simulink model "LQDG_Pitch"  (R2020a)
settings: Solver=ode3  StartTime=0.0  StopTime=inf  FixedStep=0.01  RelTol=1e-3  EnableMultiTasking=on
values from neighbouring files (symbols this model uses):
  LQDG_gain = R1_inv*B'*k1_ans    [untitled2.m]
  weighting_matrix = XOpt    [load_data.m]
undefined symbols (not defined in the file or in its folder): B1, B3, rad, s
libraries: arduinolib x5, aerolibconvert2 x4
settings Model: SILPILModeSetting=veronly  ExtModeTrigDuration=2  Creator=Ali  LastModifiedBy=Ali
settings OptimizationCC: EnhancedBackFolding=on  PassReuseOutputArgsAs=Individual arguments  ZeroExternalMemoryAtStartup=off  ZeroInternalMemoryAtStartup=off  MaxStackSize=64  OptimizeBlockOrder=speed  DifferentSizesBufferReuse=on  OptimizationCustomize=off  EfficientTunableParamExpr=on
settings DebuggingCC: ParameterTunabilityLossMsg=error
settings HardwareCC: ProdBitPerInt=16  ProdBitPerPointer=16  ProdBitPerSizeT=16  ProdBitPerPtrDiffT=16  ProdLargestAtomicFloat=None  ProdWordSize=8  ProdHWDeviceType=Atmel->AVR
settings SFSimCC: MATLABDynamicMemAlloc=off
settings RTWCC: SystemTargetFile=ert.tlc  HardwareBoard=Arduino Mega 2560  TLCOptions=-aInlineSetEventsForThisBaseRateFcn=TLC_FALSE -aSuppressMultiTaskScheduler=TLC_FALSE -aRateBasedStepFcn=1  TemplateMakefile=ert_default_tmf  Toolchain=Arduino AVR  BuildConfiguration=Faster Runs
settings CodeAppCC: ForceParamTrailComments=on  IgnoreCustomStorageClasses=off  OperatorAnnotations=on  SimulinkDataObjDesc=on  SFDataObjDesc=on  InsertBlockDesc=on
settings ERTTargetCC: SupportContinuousTime=on  SupportVariableSizeSignals=on  ExtModeStaticAllocSize=2048

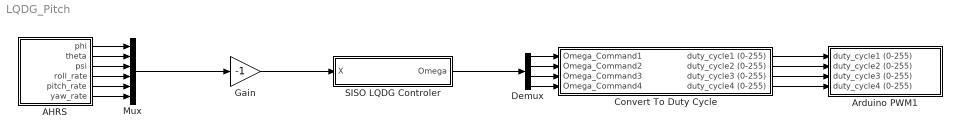
== system LQDG_Pitch ==
  AHRS : Subsystem
  Arduino PWM1 : Subsystem  mask{Motor1=8, Motor2=9, Motor3=10, Motor4=11}
      mask prompts: Motor1 "Motor 1 Pin Number"; Motor2 "Motor 2 Pin Number"; Motor3 "Motor 3 Pin Number"; Motor4 "Motor 4 Pin Number"
  Convert To Duty Cycle : Subsystem
  Demux : Demux
  Gain : Gain  Gain=-1
  Mux : Mux  Inputs=6
  SISO LQDG Controler : Subsystem
  wires:
  Convert To Duty Cycle/3(duty_cycle3 (0-255)) -> Arduino PWM1/3(duty_cycle3 (0-255))
  Convert To Duty Cycle/1(duty_cycle1 (0-255)) -> Arduino PWM1/1(duty_cycle1 (0-255))
  Convert To Duty Cycle/4(duty_cycle4 (0-255)) -> Arduino PWM1/4(duty_cycle4 (0-255))
  Convert To Duty Cycle/2(duty_cycle2 (0-255)) -> Arduino PWM1/2(duty_cycle2 (0-255))
  Demux/1 -> Convert To Duty Cycle/1(Omega_Command1)
  Demux/2 -> Convert To Duty Cycle/2(Omega_Command2)
  Demux/3 -> Convert To Duty Cycle/3(Omega_Command3)
  Demux/4 -> Convert To Duty Cycle/4(Omega_Command4)
  AHRS/1(phi) -> Mux/1
  AHRS/2(theta) -> Mux/2
  AHRS/3(psi) -> Mux/3
  AHRS/4(roll_rate) -> Mux/4
  AHRS/5(pitch_rate) -> Mux/5
  AHRS/6(yaw_rate) -> Mux/6
  Gain/1 -> SISO LQDG Controler/1(X)
  SISO LQDG Controler/1(Omega) -> Demux/1
  Mux/1 -> Gain/1

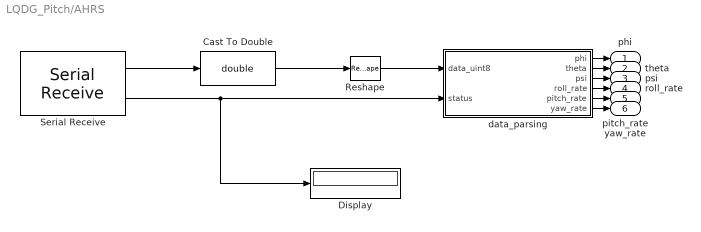
== system LQDG_Pitch/AHRS ==
  Cast To Double : DataTypeConversion  OutDataTypeStr=double
  Display : Display
  Reshape : Reshape
  Serial Receive : arduinolib/Serial Receive  isARMArch=off  portNumber=1  DataType=uint8  Datalength=32  SampleTime=0.01  showOutStatus=on  blockPlatform=arduino
      settings: SourceProductBaseCode=ARDUINO
  data_parsing : MATLAB Function  TreatAsAtomicUnit=on
  phi : Outport
  theta : Outport  Port=2
  psi : Outport  Port=3
  roll_rate : Outport  Port=4
  pitch_rate : Outport  Port=5
  yaw_rate : Outport  Port=6
  wires:
  data_parsing/2(theta) -> theta/1
  data_parsing/3(psi) -> psi/1
  data_parsing/4(roll_rate) -> roll_rate/1
  Reshape/1 -> data_parsing/1(data_uint8)
  data_parsing/1(phi) -> phi/1
  data_parsing/5(pitch_rate) -> pitch_rate/1
  Serial Receive/2 -> Display/1, data_parsing/2(status)
  data_parsing/6(yaw_rate) -> yaw_rate/1
  Cast To Double/1 -> Reshape/1
  Serial Receive/1 -> Cast To Double/1

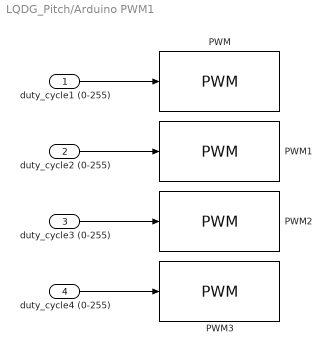
== system LQDG_Pitch/Arduino PWM1 ==
  duty_cycle1 (0-255) : Inport
  duty_cycle2 (0-255) : Inport  Port=2
  duty_cycle3 (0-255) : Inport  Port=3
  duty_cycle4 (0-255) : Inport  Port=4
  PWM : arduinolib/PWM  pinNumber=Motor1  frequencyType=Default  desiredFrequency=490.2  achievableFrequency=490.2
  PWM1 : arduinolib/PWM  pinNumber=Motor2  frequencyType=Default  desiredFrequency=490.2  achievableFrequency=490.2
  PWM2 : arduinolib/PWM  pinNumber=Motor3  frequencyType=Default  desiredFrequency=490.2  achievableFrequency=490.2
  PWM3 : arduinolib/PWM  pinNumber=Motor4  frequencyType=Default  desiredFrequency=490.2  achievableFrequency=490.2
  wires:
  duty_cycle1 (0-255)/1 -> PWM/1
  duty_cycle2 (0-255)/1 -> PWM1/1
  duty_cycle3 (0-255)/1 -> PWM2/1
  duty_cycle4 (0-255)/1 -> PWM3/1

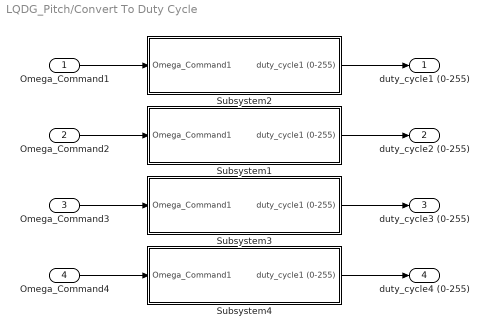
== system LQDG_Pitch/Convert To Duty Cycle ==
  Omega_Command1 : Inport
  Omega_Command2 : Inport  Port=2
  Omega_Command3 : Inport  Port=3
  Omega_Command4 : Inport  Port=4
  Subsystem1 : Subsystem
  Subsystem2 : Subsystem
  Subsystem3 : Subsystem
  Subsystem4 : Subsystem
  duty_cycle1 (0-255) : Outport
  duty_cycle2 (0-255) : Outport  Port=2
  duty_cycle3 (0-255) : Outport  Port=3
  duty_cycle4 (0-255) : Outport  Port=4
  wires:
  Subsystem1/1(duty_cycle1 (0-255)) -> duty_cycle2 (0-255)/1
  Subsystem3/1(duty_cycle1 (0-255)) -> duty_cycle3 (0-255)/1
  Subsystem4/1(duty_cycle1 (0-255)) -> duty_cycle4 (0-255)/1
  Subsystem2/1(duty_cycle1 (0-255)) -> duty_cycle1 (0-255)/1
  Omega_Command1/1 -> Subsystem2/1(Omega_Command1)
  Omega_Command4/1 -> Subsystem4/1(Omega_Command1)
  Omega_Command3/1 -> Subsystem3/1(Omega_Command1)
  Omega_Command2/1 -> Subsystem1/1(Omega_Command1)

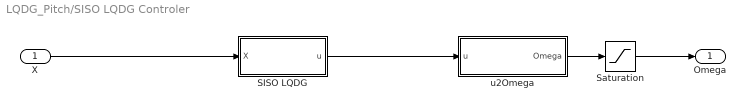
== system LQDG_Pitch/SISO LQDG Controler ==
  X : Inport
  SISO LQDG : Subsystem
  Saturation : Saturate  UpperLimit=6000*2*pi/60  LowerLimit=1500*2*pi/60
  u2Omega : Subsystem
  Omega : Outport
  wires:
  X/1 -> SISO LQDG/1(X)
  SISO LQDG/1(u) -> u2Omega/1(u)
  u2Omega/1(Omega) -> Saturation/1
  Saturation/1 -> Omega/1

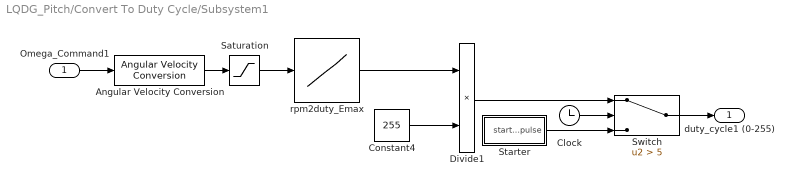
== system LQDG_Pitch/Convert To Duty Cycle/Subsystem1 ==
  Omega_Command1 : Inport
  Angular Velocity Conversion : aerolibconvert2/Angular Velocity Conversion  IU=rad/s  OU=rpm
  Clock : Clock
  Constant4 : Constant  Value=255
  Divide1 : Product  Inputs=**
  Saturation : Saturate  UpperLimit=6000  LowerLimit=1300
  Starter : Subsystem
  Switch : Switch  Criteria=u2 > Threshold  Threshold=5
  rpm2duty_Emax : Lookup_n-D  NumberOfTableDimensions=1  BreakpointsForDimension1=|  Table=|  RndMeth=Simplest  InputSameDT=on
      BreakpointsForDimension1=|
      | [1201
      | 2305
      | 3096
      | 3930
      | 4118
      | 4555
      | 5122
      | 5552
      | 5957
      | 6291
      | 6360]
      Table=|
      | [0.5
      | 0.55
      | 0.6
      | 0.65
      | 0.7
      | 0.75
      | 0.8
      | 0.85
      | 0.9
      | 0.95
      | 1]
  duty_cycle1 (0-255) : Outport
  wires:
  Divide1/1 -> Switch/1
  Switch/1 -> duty_cycle1 (0-255)/1
  Clock/1 -> Switch/2
  Starter/1(start_pulse) -> Switch/3
  Angular Velocity Conversion/1 -> Saturation/1
  Constant4/1 -> Divide1/2
  Omega_Command1/1 -> Angular Velocity Conversion/1
  rpm2duty_Emax/1 -> Divide1/1
  Saturation/1 -> rpm2duty_Emax/1

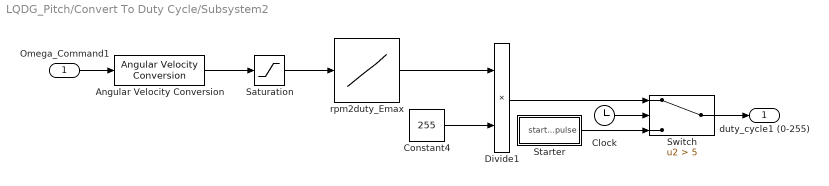
== system LQDG_Pitch/Convert To Duty Cycle/Subsystem2 ==
  Omega_Command1 : Inport
  Angular Velocity Conversion : aerolibconvert2/Angular Velocity Conversion  IU=rad/s  OU=rpm
  Clock : Clock
  Constant4 : Constant  Value=255
  Divide1 : Product  Inputs=**
  Saturation : Saturate  UpperLimit=6000  LowerLimit=1300
  Starter : Subsystem
  Switch : Switch  Criteria=u2 > Threshold  Threshold=5
  rpm2duty_Emax : Lookup_n-D  NumberOfTableDimensions=1  BreakpointsForDimension1=|  Table=|  RndMeth=Simplest  InputSameDT=on
      BreakpointsForDimension1=|
      | [1201
      | 2305
      | 3096
      | 3930
      | 4118
      | 4555
      | 5122
      | 5552
      | 5957
      | 6291
      | 6360]
      Table=|
      | [0.5
      | 0.55
      | 0.6
      | 0.65
      | 0.7
      | 0.75
      | 0.8
      | 0.85
      | 0.9
      | 0.95
      | 1]
  duty_cycle1 (0-255) : Outport
  wires:
  Omega_Command1/1 -> Angular Velocity Conversion/1
  Constant4/1 -> Divide1/2
  Angular Velocity Conversion/1 -> Saturation/1
  Starter/1(start_pulse) -> Switch/3
  Clock/1 -> Switch/2
  Switch/1 -> duty_cycle1 (0-255)/1
  Divide1/1 -> Switch/1
  rpm2duty_Emax/1 -> Divide1/1
  Saturation/1 -> rpm2duty_Emax/1

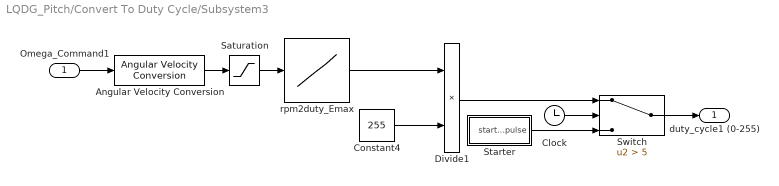
== system LQDG_Pitch/Convert To Duty Cycle/Subsystem3 ==
  Omega_Command1 : Inport
  Angular Velocity Conversion : aerolibconvert2/Angular Velocity Conversion  IU=rad/s  OU=rpm
  Clock : Clock
  Constant4 : Constant  Value=255
  Divide1 : Product  Inputs=**
  Saturation : Saturate  UpperLimit=6000  LowerLimit=1300
  Starter : Subsystem
  Switch : Switch  Criteria=u2 > Threshold  Threshold=5
  rpm2duty_Emax : Lookup_n-D  NumberOfTableDimensions=1  BreakpointsForDimension1=|  Table=|  RndMeth=Simplest  InputSameDT=on
      BreakpointsForDimension1=|
      | [1201
      | 2305
      | 3096
      | 3930
      | 4118
      | 4555
      | 5122
      | 5552
      | 5957
      | 6291
      | 6360]
      Table=|
      | [0.5
      | 0.55
      | 0.6
      | 0.65
      | 0.7
      | 0.75
      | 0.8
      | 0.85
      | 0.9
      | 0.95
      | 1]
  duty_cycle1 (0-255) : Outport
  wires:
  Omega_Command1/1 -> Angular Velocity Conversion/1
  Constant4/1 -> Divide1/2
  Angular Velocity Conversion/1 -> Saturation/1
  Starter/1(start_pulse) -> Switch/3
  Clock/1 -> Switch/2
  Switch/1 -> duty_cycle1 (0-255)/1
  Divide1/1 -> Switch/1
  rpm2duty_Emax/1 -> Divide1/1
  Saturation/1 -> rpm2duty_Emax/1

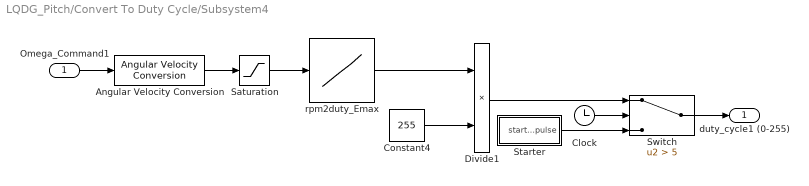
== system LQDG_Pitch/Convert To Duty Cycle/Subsystem4 ==
  Omega_Command1 : Inport
  Angular Velocity Conversion : aerolibconvert2/Angular Velocity Conversion  IU=rad/s  OU=rpm
  Clock : Clock
  Constant4 : Constant  Value=255
  Divide1 : Product  Inputs=**
  Saturation : Saturate  UpperLimit=6000  LowerLimit=1300
  Starter : Subsystem
  Switch : Switch  Criteria=u2 > Threshold  Threshold=5
  rpm2duty_Emax : Lookup_n-D  NumberOfTableDimensions=1  BreakpointsForDimension1=|  Table=|  RndMeth=Simplest  InputSameDT=on
      BreakpointsForDimension1=|
      | [1201
      | 2305
      | 3096
      | 3930
      | 4118
      | 4555
      | 5122
      | 5552
      | 5957
      | 6291
      | 6360]
      Table=|
      | [0.5
      | 0.55
      | 0.6
      | 0.65
      | 0.7
      | 0.75
      | 0.8
      | 0.85
      | 0.9
      | 0.95
      | 1]
  duty_cycle1 (0-255) : Outport
  wires:
  Divide1/1 -> Switch/1
  Switch/1 -> duty_cycle1 (0-255)/1
  Clock/1 -> Switch/2
  Starter/1(start_pulse) -> Switch/3
  Angular Velocity Conversion/1 -> Saturation/1
  Constant4/1 -> Divide1/2
  Omega_Command1/1 -> Angular Velocity Conversion/1
  rpm2duty_Emax/1 -> Divide1/1
  Saturation/1 -> rpm2duty_Emax/1

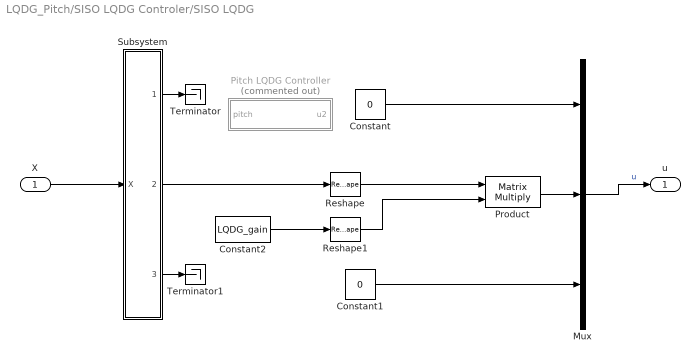
== system LQDG_Pitch/SISO LQDG Controler/SISO LQDG ==
  X : Inport
  Constant : Constant  Value=0
  Constant1 : Constant  Value=0
  Constant2 : Constant  Value=LQDG_gain
  Mux : Mux  Inputs=3
  Pitch LQDG Controller : Subsystem  Commented=on
  Product : Product  Multiplication=Matrix(*)
  Reshape : Reshape  OutputDimensionality=Row vector (2-D)
  Reshape1 : Reshape  OutputDimensionality=Column vector (2-D)
  Subsystem : Subsystem
  Terminator : Terminator
  Terminator1 : Terminator
  u : Outport
  wires:
  Mux/1 -> u/1  "u"
  X/1 -> Subsystem/1(X)
  Subsystem/1(roll) -> Terminator/1
  Constant/1 -> Mux/1
  Subsystem/3(yaw) -> Terminator1/1
  Constant1/1 -> Mux/3
  Subsystem/2(pitch) -> Reshape/1
  Constant2/1 -> Reshape1/1
  Reshape/1 -> Product/1
  Product/1 -> Mux/2
  Reshape1/1 -> Product/2

== system LQDG_Pitch/SISO LQDG Controler/u2Omega ==
  u : Inport
  MATLAB Function1 : MATLAB Function  TreatAsAtomicUnit=on
  Mux1 : Mux
  Omega : Outport
  wires:
  Mux1/1 -> Omega/1
  MATLAB Function1/2(omega_2) -> Mux1/2
  u/1 -> MATLAB Function1/1(u)
  MATLAB Function1/3(omega_3) -> Mux1/3
  MATLAB Function1/1(omega_1) -> Mux1/1
  MATLAB Function1/4(omega_4) -> Mux1/4

== system LQDG_Pitch/Convert To Duty Cycle/Subsystem1/Starter ==
  Add : Sum
  Step : Step  After=140
  Step1 : Step  Time=2  After=-30
  start_pulse : Outport
  wires:
  Add/1 -> start_pulse/1
  Step/1 -> Add/1
  Step1/1 -> Add/2

== system LQDG_Pitch/Convert To Duty Cycle/Subsystem2/Starter ==
  Add : Sum
  Step : Step  After=140
  Step1 : Step  Time=2  After=-30
  start_pulse : Outport
  wires:
  Add/1 -> start_pulse/1
  Step/1 -> Add/1
  Step1/1 -> Add/2

== system LQDG_Pitch/Convert To Duty Cycle/Subsystem3/Starter ==
  Add : Sum
  Step : Step  After=140
  Step1 : Step  Time=2  After=-30
  start_pulse : Outport
  wires:
  Add/1 -> start_pulse/1
  Step/1 -> Add/1
  Step1/1 -> Add/2

== system LQDG_Pitch/Convert To Duty Cycle/Subsystem4/Starter ==
  Add : Sum
  Step : Step  After=140
  Step1 : Step  Time=2  After=-30
  start_pulse : Outport
  wires:
  Add/1 -> start_pulse/1
  Step/1 -> Add/1
  Step1/1 -> Add/2

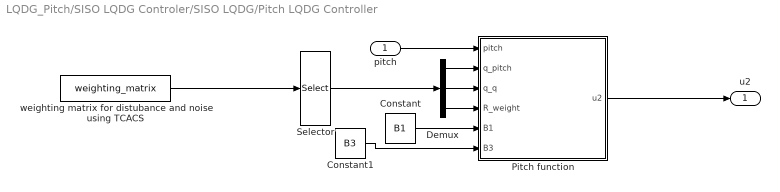
== system LQDG_Pitch/SISO LQDG Controler/SISO LQDG/Pitch LQDG Controller ==
  pitch : Inport
  Constant : Constant  Value=B1
  Constant1 : Constant  Value=B3
  Demux : Demux  Outputs=3
  Pitch function : MATLAB Function  TreatAsAtomicUnit=on
  Selector : Selector  InputPortWidth=5  IndexOptions=Index vector (dialog)  Indices=[1 3 5]  OutputSizes=1
  weighting matrix for distubance and noise using TCACS : Constant  Value=weighting_matrix
  u2 : Outport
  wires:
  Pitch function/1(u2) -> u2/1
  Demux/1 -> Pitch function/2(q_pitch)
  Demux/3 -> Pitch function/4(R_weight)
  Selector/1 -> Demux/1
  Demux/2 -> Pitch function/3(q_q)
  weighting matrix for distubance and noise using TCACS/1 -> Selector/1
  pitch/1 -> Pitch function/1(pitch)
  Constant/1 -> Pitch function/5(B1)
  Constant1/1 -> Pitch function/6(B3)

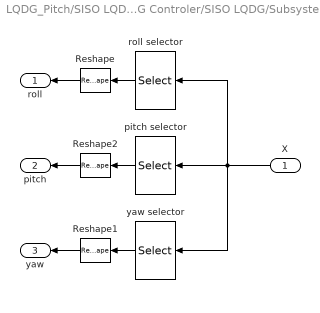
== system LQDG_Pitch/SISO LQDG Controler/SISO LQDG/Subsystem ==
  X : Inport
  Reshape : Reshape  OutputDimensionality=Column vector (2-D)
  Reshape1 : Reshape  OutputDimensionality=Column vector (2-D)
  Reshape2 : Reshape  OutputDimensionality=Column vector (2-D)
  pitch selector : Selector  InputPortWidth=6  IndexOptions=Index vector (dialog)  Indices=[2 5]  OutputSizes=1
  roll selector : Selector  InputPortWidth=6  IndexOptions=Index vector (dialog)  Indices=[1 4]  OutputSizes=1
  yaw selector : Selector  InputPortWidth=6  IndexOptions=Index vector (dialog)  Indices=[3 6]  OutputSizes=1
  roll : Outport
  pitch : Outport  Port=2
  yaw : Outport  Port=3
  wires:
  X/1 -> yaw selector/1, roll selector/1, pitch selector/1
  roll selector/1 -> Reshape/1
  pitch selector/1 -> Reshape2/1
  yaw selector/1 -> Reshape1/1
  Reshape/1 -> roll/1
  Reshape2/1 -> pitch/1
  Reshape1/1 -> yaw/1

== matlab function LQDG_Pitch/SISO LQDG Controler/u2Omega/MATLAB Function1 ==
  data: u input size=3; omega_1 output size=1; omega_2 output size=1; omega_3 output size=1; omega_4 output size=1
function [omega_1, omega_2, omega_3, omega_4] = fcn(u)
u1 = u(1);
u2 = u(2);
u3 = u(3);
% control effort
u4 = ones(1, length(u1)) * 4 * rpm2rad_sec(2000)^2;
% calculate omega
if (u4 + u3 + 2 * u2) / 4 > 0
    omega_1 = sqrt((u4 + u3 + 2 * u2) / 4);
else
    omega_1 = 0;
end
if (u4 + u3 - 2 * u2) / 4 > 0
    omega_3 = sqrt((u4 + u3 - 2 * u2) / 4);
else
    omega_3 = 0;
end
if (u4 - u3 + 2 * u1) / 4 > 0
    omega_2 = sqrt((u4 - u3 + 2 * u1) / 4);
else
    omega_2 = 0;
end
if (u4 - u3 - 2 * u1) / 4 > 0
    omega_4 = sqrt((u4 - u3 - 2 * u1) / 4);
else
    omega_4 = 0;
end
end
%% functions
% rpm to rad/sec
function rad = rpm2rad_sec(rpm)
rad = rpm / 60 * 2 * pi;
end

== matlab function LQDG_Pitch/AHRS/data_parsing ==
  data: phi output size=1; data_uint8 input size=32; theta output size=1; psi output size=1; roll_rate output size=1; pitch_rate output size=1; yaw_rate output size=1; status input
function [phi,theta,psi,roll_rate,pitch_rate,yaw_rate] = fcn(data_uint8, status)
persistent stepp check_sum...
    phi_p theta_p psi_p roll_rate_p pitch_rate_p yaw_rate_p...
    phi_last theta_last psi_last roll_rate_last pitch_rate_last yaw_rate_last;
%% Initialize
if isempty(stepp)
    stepp=0;
    check_sum=0;
    phi_p=0;
    theta_p=0;
    psi_p=0;
    roll_rate_p=0;
    pitch_rate_p=0;
    yaw_rate_p=0;
    phi_last=0;
    theta_last=0;
    psi_last=0;
    roll_rate_last=0;
    pitch_rate_last=0;
    yaw_rate_last=0;
end
angle_scale=.0109863;  % 1/91.0222
rate_scale=1/16;
%% Check Each Byte
if status
    for i = 1:length(data_uint8)
        if (data_uint8(i)==115 && stepp==0)
            stepp=1;
            check_sum=data_uint8(i);
        elseif(stepp==1 && data_uint8(i)==110)
            stepp=stepp+1;
            check_sum=check_sum+data_uint8(i);
        elseif(stepp==2 && data_uint8(i)==112)
            stepp=stepp+1;
            check_sum=check_sum+data_uint8(i);
        elseif(stepp==3 && data_uint8(i)==212)
            stepp=stepp+1;
            check_sum=check_sum+data_uint8(i);
        elseif(stepp==4 && data_uint8(i)==112)
            stepp=stepp+1;
            check_sum=check_sum+data_uint8(i);
        elseif(stepp==5)
            phi_p=data_uint8(i)*256;
            stepp=stepp+1;
            check_sum=check_sum+data_uint8(i);
        elseif(stepp==6)
            phi_p=phi_p+data_uint8(i);
            stepp=stepp+1;
            check_sum=check_sum+data_uint8(i);
        elseif(stepp==7)
            theta_p=data_uint8(i)*256;
            stepp=stepp+1;
            check_sum=check_sum+data_uint8(i);
        elseif(stepp==8)
            theta_p=theta_p+data_uint8(i);
            stepp=stepp+1;
            check_sum=check_sum+data_uint8(i);
        elseif(stepp==9)
            psi_p=data_uint8(i)*256;
            stepp=stepp+1;
            check_sum=check_sum+data_uint8(i);
        elseif(stepp==10)
            psi_p=psi_p+data_uint8(i);
            stepp=stepp+1;
            check_sum=check_sum+data_uint8(i);
        elseif(stepp==11 || stepp==12)
            if(data_uint8(i)==0)
                stepp=stepp+1;
            else
                stepp=0;
            end
        elseif(stepp==13)
            roll_rate_p=data_uint8(i)*256;
            stepp=stepp+1;
            check_sum=check_sum+data_uint8(i);
        elseif(stepp==14)
            roll_rate_p=roll_rate_p+data_uint8(i);
            stepp=stepp+1;
            check_sum=check_sum+data_uint8(i);
        elseif(stepp==15)
            pitch_rate_p=data_uint8(i)*256;
            stepp=stepp+1;
            check_sum=check_sum+data_uint8(i);
        elseif(stepp==16)
            pitch_rate_p=pitch_rate_p+data_uint8(i);
            stepp=stepp+1;
            check_sum=check_sum+data_uint8(i);
        elseif(stepp==17)
            yaw_rate_p=data_uint8(i)*256;
            stepp=stepp+1;
            check_sum=check_sum+data_uint8(i);
        elseif(stepp==18)
            yaw_rate_p=yaw_rate_p+data_uint8(i);
            stepp=stepp+1;
            check_sum=check_sum+data_uint8(i);
        elseif(stepp==19 || stepp==20)
            if(data_uint8(i)==0)
                stepp=stepp+1;
            else
                stepp=0;
            end
        elseif(stepp==21 || stepp==22 || stepp==23 || stepp==24)
            stepp=stepp+1;
            check_sum=check_sum+data_uint8(i);
        elseif(stepp==25)
            if (floor(check_sum/256)==data_uint8(i))
                stepp=stepp+1;
            else
                stepp=0;
            end
        elseif(stepp==26)
            if(mod(check_sum,256)==data_uint8(i))
                phi_last=double(typecast(uint16(phi_p), 'int16'))*angle_scale;
                if mod(phi_last,360)>180
                    phi_last=mod(phi_last,360)-360;
                else
                    phi_last=mod(phi_last,360);
                end
                theta_last=double(typecast(uint16(theta_p), 'int16'))*angle_scale;
                if mod(theta_last,360)>180
                    theta_last=mod(theta_last,360)-360;
                else
                    theta_last=mod(theta_last,360);
                end
                psi_last=double(typecast(uint16(psi_p), 'int16'))*angle_scale;
                if mod(psi_last,360)>180
                    psi_last=mod(psi_last,360)-360;
                else
                    psi_last=mod(psi_last,360);
                end
                roll_rate_last=double(typecast(uint16(roll_rate_p), 'int16'))*rate_scale;
                if mod(roll_rate_last,360)>180
                    roll_rate_last=mod(roll_rate_last,360)-360;
                else
                    roll_rate_last=mod(roll_rate_last,360);
                end
                pitch_rate_last=double(typecast(uint16(pitch_rate_p), 'int16'))*rate_scale;
                if mod(pitch_rate_last,360)>180
                    pitch_rate_last=mod(pitch_rate_last,360)-360;
                else
                    pitch_rate_last=mod(pitch_rate_last,360);
                end
                yaw_rate_last=double(typecast(uint16(yaw_rate_p), 'int16'))*rate_scale;
                if mod(yaw_rate_last,360)>180
                    yaw_rate_last=mod(yaw_rate_last,360)-360;
                else
                    yaw_rate_last=mod(yaw_rate_last,360);
                end
            end
            stepp=0;
        end
    end
end

%% Assign Last True Data to Output
phi=phi_last;
theta=theta_last;
psi=psi_last;
roll_rate=roll_rate_last;
pitch_rate=pitch_rate_last;
yaw_rate=yaw_rate_last;

== matlab function LQDG_Pitch/SISO LQDG Controler/SISO LQDG/Pitch LQDG Controller/Pitch function ==
  data: pitch input; u2 output; q_pitch input; q_q input; R_weight input; B1 input; B3 input
function u2 = fcn(pitch, q_pitch, q_q, R_weight, B1, B3)
% QuadConstants;
% QuadConstants;
%%% constans %%%
% Distance between rotor center to quad center (m)
% d_cg = 0.295;
% Distance between D point to quad center (m)
% h_cg = 0.0078;
% Thrust factor (non dimensional)
% b = 1.10794e-5;
% Rotor torque drag factor (non dimensional)
% d = 3.2e-6;
% Total mass (kg)
% m_tot = 1.774;
% Quad Moment of inertia respect to axix X Body (kg.m^2)
% J_xx = 0.0297598;
% Quad Moment of inertia respect to axix Y Body (kg.m^2)
% J_yy = 0.0298565;
% Quad Moment of inertia respect to axix Y Body (kg.m^2)
% J_zz = 0.058510;
% Quad blade Moment (kg.m^2)
% J_R = 4.439e-5;
% Mass on X axis bearing (kg)
% m1 = 1.272;
% Mass on Y axis bearing (kg)
% m2 = 1.074;
% Mass on Z axis bearing (kg)
% m3 = 1.693;
% Bearing radius in X axix (m)
% r_x = 0.01;
% Bearing radius in Y axix (m)
% r_y = 0.01;
% Bearing radius in Z axix (m)
% r_z = 0.025;
% Static bearing friction (non dimensional)
% miu_s = 0.003;
% Dynamic bearing friction (non dimensional)
% miu_k = 0.002;
% Motor constant (non dimensional)
% tau = 0.15;
% Delay of motor (sec)
% T_d = 0.02;
% Gravity force (m/s^2)
% g = 9.81;
% A Constants
% A1 = (h_cg * g * m_tot) / (m_tot * h_cg^2 + J_xx);
% A2 = (2*m_tot * h_cg^2 + J_yy -J_zz) / (m_tot * h_cg^2 + J_xx);
% A3 = (b * d_cg) / (m_tot * h_cg^2 + J_xx);
% A4 = (J_R) / (m_tot * h_cg^2 + J_xx);
% A5 = (m1 * g * miu_k * r_x) / (m_tot * h_cg^2 + J_xx);
% B Constants
% B1 = (h_cg * g * m_tot) / (m_tot * h_cg^2 + J_yy);
% B2 = (-2*m_tot * h_cg^2 - J_xx + J_zz) / (m_tot * h_cg^2 + J_yy);
% B3 = (b * d_cg) / (m_tot * h_cg^2 + J_yy);
% B4 = (-J_R) / (m_tot * h_cg^2 + J_yy);
% B5 = (m2 * g * miu_k * r_y) / (m_tot * h_cg^2 + J_yy);
% C Constants
% C1 = (J_xx - J_yy) / (J_zz);
% C2 = (d) / (J_zz);
% C3 = (m3 * g * miu_k * r_z) / (J_zz);
% omega for linearzation 2000 RPM
% Omega = 2000 / 60 * 2 * pi;

x2     = pitch(1);
A22    = 0; %da2dx2
A25    = 1; %da2dx5
A52    = B1 * cos(x2); %da5dx2
A55    = 0; %da5dx5

A      = [A22, A25 ;
          A52, A55];
B      = [0  ;
          B3];
a      = A(2);
b      = B(2);

q1     = 10^q_pitch;
q2     = 10^q_q;
R1     = 1;
R2     = 10^R_weight;
R1_inv = R1^-1;
R2_inv = R2^-1;
k1_ans = zeros(2, 2);
k2_ans = zeros(2, 2);

% algebraic_riccati = K * A + A' * K - K * B * R^-1 * B' * K + Q;
% first equation q1 + 2*a*k12 - (b^2*k12^2)/R = 0
% Ans1 K12 = -m*(k + (k^2 + Q11)^(1/2))
% Ans2 K12 = -m*(k - (k^2 + Q11)^(1/2))
valid_ans = false; % answer validation for statble system
k12_1 = zeros(1, 2);
k12_2 = zeros(1, 2);
k12_1(1) =   (R1*R2*a + R1*b^2*((R1*R2*(R1*R2*a^2 + R1*b^2*q1 + R2*b^2*q1))/(b^4*(R1 + R2)^2))^(1/2) + R2*b^2*((R1*R2*(R1*R2*a^2 + R1*b^2*q1 + R2*b^2*q1))/(b^4*(R1 + R2)^2))^(1/2))/(R1*b^2 + R2*b^2);
k12_1(2) =  -(R1*b^2*((R1*R2*(R1*R2*a^2 + R1*b^2*q1 + R2*b^2*q1))/(b^4*(R1 + R2)^2))^(1/2) - R1*R2*a + R2*b^2*((R1*R2*(R1*R2*a^2 + R1*b^2*q1 + R2*b^2*q1))/(b^4*(R1 + R2)^2))^(1/2))/(R1*b^2 + R2*b^2);
k12_2(1) =  (R1*R2*a + R1*b^2*((R1*R2*(R1*R2*a^2 + R1*b^2*q1 + R2*b^2*q1))/(b^4*(R1 + R2)^2))^(1/2) + R2*b^2*((R1*R2*(R1*R2*a^2 + R1*b^2*q1 + R2*b^2*q1))/(b^4*(R1 + R2)^2))^(1/2))/(R1*b^2 + R2*b^2);
for i = 1:length(k12_1)
    % Second equation 
    % 1 (b^2*k22_1^2)/R1 + (k22_2*b^2*k22_1)/R2 - 2*k12_1 - q2 = 0
    % 2 (b^2*k22_2^2)/R2 + (k22_1*b^2*k22_2)/R1 - 2*k12_2 - q2
    % Ans1 K22_1 =  -((2*k12_1 + q2)*((R1*R2*
    % (2*k12_2 + q2)^2)/(b^2*(2*R1*k12_2 + 2*R2*k12_1 + R1*q2 + R2*q2)))
    % ^(1/2))/(2*k12_2 + q2)
    
    % Ans2 K22_1 = ((2*k12_1 + q2)*((R1*R2*(2*k12_2 + q2)^2)
    % /(b^2*(2*R1*k12_2 + 2*R2*k12_1 + R1*q2 + R2*q2)))^(1/2))/(2*k12_2 + q2)
    
    % Ans1 K22_2 =  -((R1*R2*(2*k12_2 + q2)^2)/(b^2*
    % (2*R1*k12_2 + 2*R2*k12_1 + R1*q2 + R2*q2)))^(1/2)

    % Ans1 K22_2 = ((R1*R2*(2*k12_2 + q2)^2)/
    % (b^2*(2*R1*k12_2 + 2*R2*k12_1 + R1*q2 + R2*q2)))^(1/2)
    
    k22_1 = zeros(1, 2);
    k22_2 = zeros(1, 2);
    valid22 = [true; true]; % for validation in complex number
    if ((R1*R2*(2*k12_2(i) + q2)^2)/(b^2*(2*R1*k12_2(i) + 2*R2*k12_1(i) + R1*q2 + R2*q2))) < 0 
        valid22(i) = false;
    else
        k22_1(1) = -((2*k12_1(i) + q2)*((R1*R2*(2*k12_2(i) + q2)^2)/(b^2*(2*R1*k12_2(i) + 2*R2*k12_1(i) + R1*q2 + R2*q2)))^(1/2))/(2*k12_2(i) + q2);
    end
    if ((R1*R2*(2*k12_2(i) + q2)^2)/(b^2*(2*R1*k12_2(i) + 2*R2*k12_1(i) + R1*q2 + R2*q2))) < 0
        valid22(i) = false;
    else
        k22_1(2) =  ((2*k12_1(i) + q2)*((R1*R2*(2*k12_2(i) + q2)^2)/(b^2*(2*R1*k12_2(i) + 2*R2*k12_1(i) + R1*q2 + R2*q2)))^(1/2))/(2*k12_2(i) + q2);
    end
    if ((R1*R2*(2*k12_2(i) + q2)^2)/(b^2*(2*R1*k12_2(i) + 2*R2*k12_1(i) + R1*q2 + R2*q2))) < 0
        valid22(i) = false;
    else
        k22_2(1) = -((R1*R2*(2*k12_2(i) + q2)^2)/(b^2*(2*R1*k12_2(i) + 2*R2*k12_1(i) + R1*q2 + R2*q2)))^(1/2);
        k22_2(2) =  ((R1*R2*(2*k12_2(i) + q2)^2)/(b^2*(2*R1*k12_2(i) + 2*R2*k12_1(i) + R1*q2 + R2*q2)))^(1/2);
    end
    for j = 1:length(k22_1)
        if valid22(i) == false
            continue
        end
        % Last equation 
        % 1 (b^2*k12_1*k22_1)/R1 - a*k22_1 - k11_1 + (b^2*k12_2*k22_1)/R2
        % Ans k11_1 = (b^2*k12_1*k22_1)/R1 - a*k22_1 + (b^2*k12_2*k22_1)/R2
        % Ans k11_2 = (b^2*k12_1*k22_1)/R1 - a*k22_1 + (b^2*k12_2*k22_1)/R2
        k11_1 = (b^2*k12_1(i)*k22_1(j))/R1 - a*k22_1(j) + (b^2*k12_2(i)*k22_1(j))/R2;
        k11_2 = (b^2*k12_1(i)*k22_2(j))/R1 - a*k22_2(j) + (b^2*k12_2(i)*k22_2(j))/R2;
        temp_K_1 = zeros(2, 2);
        temp_K_1(1, 1) = k11_1;
        temp_K_1(1, 2) = k12_1(i);
        temp_K_1(2, 1) = k12_1(i);
        temp_K_1(2, 2) = k22_1(j);
        temp_K_2 = zeros(2, 2);
        temp_K_2(1, 1) = k11_2;
        temp_K_2(1, 2) = k12_2(i);
        temp_K_2(2, 1) = k12_2(i);
        temp_K_2(2, 2) = k22_2(j);
        if all(eig(A + (-B*R1_inv*B'*temp_K_1 - B*R2_inv*B'*temp_K_2)) < 0)
            k1_ans = temp_K_1;
            k2_ans = temp_K_2;
            valid_ans = true;
            break;
        end
        if valid_ans == true
            break;
        end
    end
    if valid_ans == true
        break;
    end
end

u2 = (R1_inv*B'*k1_ans + R2_inv*B'*k2_ans) *pitch;
